simulink model "SS_ServoFire"  (R2019b)
settings: Solver=VariableStepAuto  StartTime=0.0  StopTime=60.0  FixedStep=0.00000001  RelTol=1e-3
undefined symbols (not defined in the file): __PRM__SERIALIZED__DATA__, SubsystemReferenceBlock
settings Model: Creator=toons  LastModifiedBy=toons
settings SolverCC: ZeroCrossAlgorithm=Adaptive
settings DataIOCC: ExternalInput=[input1, input2]  ReturnWorkspaceOutputs=off
settings DebuggingCC: IgnoredZcDiagnostic=none  ArithmeticOperatorsInVariantConditions=warning
settings SFSimCC: CustomCodeUndefinedFunction=UseInterfaceOnly

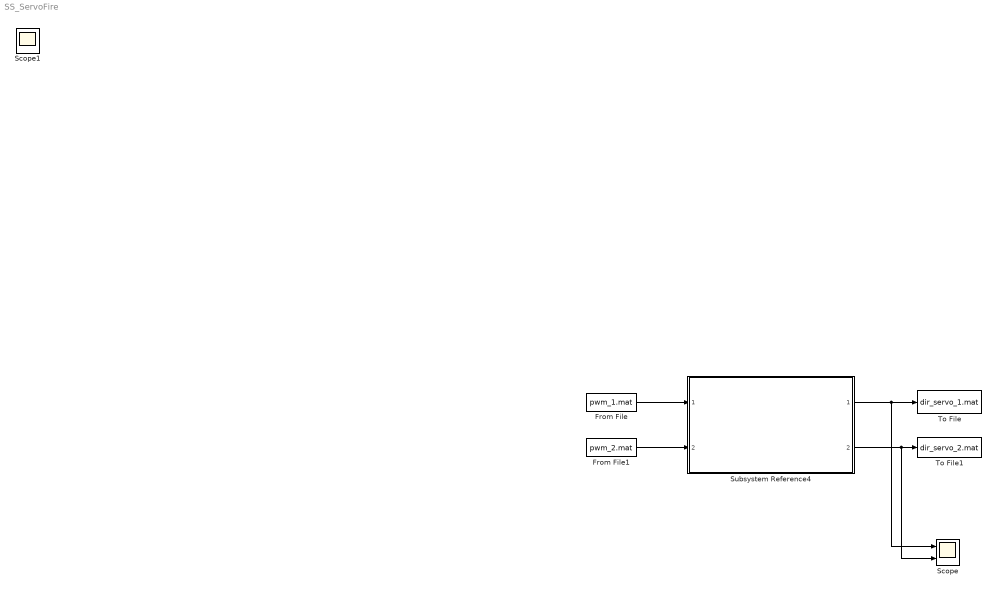
== system SS_ServoFire ==
  From File : FromFile  FileName=pwm_1.mat  SampleTime=0  ExtrapolationBeforeFirstDataPoint=Ground value  InterpolationWithinTimeRange=Zero order hold  ExtrapolationAfterLastDataPoint=Ground value
  From File1 : FromFile  FileName=pwm_2.mat  SampleTime=0  ExtrapolationBeforeFirstDataPoint=Ground value  InterpolationWithinTimeRange=Zero order hold  ExtrapolationAfterLastDataPoint=Ground value
  Scope : Scope  NumInputPorts=2
  Subsystem Reference4 : Subsystem  BlockKeywords=__PRM__SERIALIZED__DATA__:SubsystemReferenceBlock  ReferencedSubsystem=ServoSimulation
  To File : ToFile  Filename=dir_servo_1.mat  SaveFormat=Timeseries
  To File1 : ToFile  Filename=dir_servo_2.mat  SaveFormat=Timeseries
  Scope1 : Scope
  wires:
  From File/1 -> Subsystem Reference4/1
  From File1/1 -> Subsystem Reference4/2
  Subsystem Reference4/1 -> Scope/1, To File/1
  Subsystem Reference4/2 -> To File1/1, Scope/2
